simulink model "L2pend_self"  (R2022a)
settings: Solver=ode3  StartTime=0.0  StopTime=10.0  FixedStep=0.01  RelTol=1e-3
undefined symbols (not defined in the file): A, B, C, D, ics, x0
libraries: simulink_extras x2
settings Model: Creator=Dizzy  LastModifiedBy=Dizzy

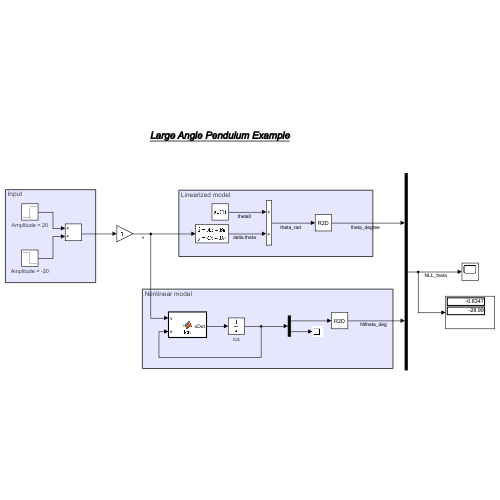
[thumbnail: Simulink's stored preview of the top-level diagram]
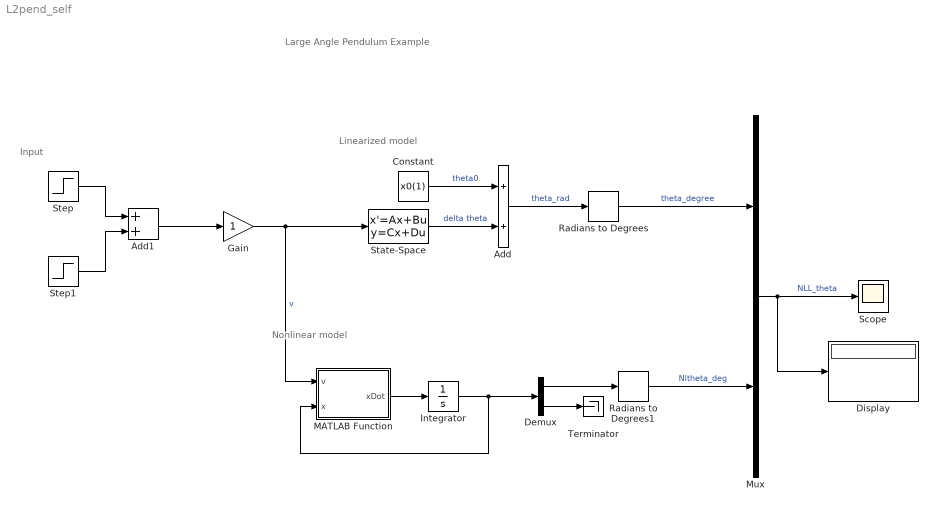
== system L2pend_self ==
  note: Large Angle Pendulum Example
  note: Input
  note: Nonlinear model
  note: Linearized model
  Add : Sum
  Add1 : Sum
  Constant : Constant  Value=x0(1)
  Demux : Demux  Outputs=[1 2]
  Display : Display
  Gain : Gain
  Integrator : Integrator  InitialCondition=ics
      settings: AttributesFormatString=%<InitialCondition>
  MATLAB Function : MATLAB Function  TreatAsAtomicUnit=on
  Mux : Mux  Inputs=2
  Radians to Degrees : simulink_extras/Transformations/Radians to Degrees
  Radians to Degrees1 : simulink_extras/Transformations/Radians to Degrees
  Scope : Scope
  State-Space : StateSpace  A=A  B=B  C=C  D=D  InitialCondition=[0;0;0]
  Step : Step  After=20  SampleTime=0
      settings: AttributesFormatString=Amplitude = %<After>
  Step1 : Step  Time=2  After=-20  SampleTime=0
      settings: AttributesFormatString=Amplitude = %<After>
  Terminator : Terminator
  wires:
  Constant/1 -> Add/1  "theta0"
  State-Space/1 -> Add/2  "delta theta"
  Add/1 -> Radians to Degrees/1  "theta_rad"
  Radians to Degrees/1 -> Mux/1  "theta_degree"
  MATLAB Function/1(xDot) -> Integrator/1
  Integrator/1 -> Demux/1, MATLAB Function/2(x)
  Radians to Degrees1/1 -> Mux/2  "Nltheta_deg"
  Step/1 -> Add1/1
  Step1/1 -> Add1/2
  Add1/1 -> Gain/1
  Gain/1 -> MATLAB Function/1(v), State-Space/1  "v"
  Mux/1 -> Display/1, Scope/1  "NLL_theta"
  Demux/1 -> Radians to Degrees1/1
  Demux/2 -> Terminator/1

== matlab function L2pend_self/MATLAB Function ==
  data: v input size=1; x input size=3; xDot output size=3
function xDot = fcn(v, x)

g = 10; % (m/s^2)
L =  2; % (m)
m =  1; % (kg)
kt = .5; % (N/A)
kb = .5; % V-s
ra = 1; % (ohm)
la = .1; % (H)

% Lumped parameters
a1 = -g/L;
a2 = kt/m/L/L;
a3 = -ra/la;
a4 = -kb/la;
b1 = 1/la;

% Grab memory for the output
xDot = zeros(3,1);

% Create f of x' = f(x,u)
xDot(1) = x(2);
xDot(2) = a1*sin(x(1)) + a2*x(3);
xDot(3) = a3*x(3) + a4*x(2) + b1*v(1);
